simulink model "frmBuilder_sl_interactions_with_sfun_wrapper_for_testing"  (R2017b)
settings: Solver=FixedStepAuto  StartTime=0.0  StopTime=10.0  RelTol=1e-3  EnableMultiTasking=on
settings Model: Creator=na364  LastModifiedBy=na364
settings DataIOCC: LimitDataPoints=on
settings OptimizationCC: LifeSpan=inf
settings DebuggingCC: AllowSymbolicDim=off  SFUnexpectedBacktrackingDiag=warning  SFNoUnconditionalDefaultTransitionDiag=warning  SFExecutionAtInitializationDiag=none
settings ModelReferenceCC: ModelReferenceNumInstancesAllowed=Single  PropagateSignalLabelsOutOfModel=off
settings CodeAppCC: StateflowObjectComments=on
settings GRTTargetCC: TargetLangStandard=C89/C90 (ANSI)
settings ConfigComp: CovMetricSettings=dw  CovHtmlReporting=on  CovSaveCumulativeToWorkspaceVar=on  CovSaveSingleToWorkspaceVar=on  CovExternalEMLEnable=off

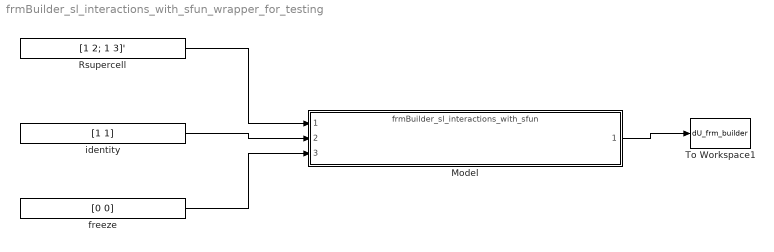
== system frmBuilder_sl_interactions_with_sfun_wrapper_for_testing ==
  Model : ModelReference  ModelNameDialog=frmBuilder_sl_interactions_with_sfun.slx  SimulationMode=Normal  ModelReferenceVersion=1.340
  Rsupercell : Constant  Value=[1 2; 1 3]'
  To Workspace1 : ToWorkspace  VariableName=dU_frm_builder  SampleTime=-1
  freeze : Constant  Value=[0 0]
  identity : Constant  Value=[1 1]
  wires:
  freeze/1 -> Model/3
  identity/1 -> Model/2
  Rsupercell/1 -> Model/1
  Model/1 -> To Workspace1/1
